simulink model "Final_Project_EEM_Particle_SIM"  (R2020a)
settings: Solver=ode45  StartTime=0  StopTime=t_runtime  FixedStep=clockt/4  RelTol=1e-3  AbsTol=1e-6
PreLoadFcn:
  | run('Final_Project_EEM_SIM_init_params.m');
StopFcn:
  | run('Particle_Simulation_Run_Plots_EEM.m');
undefined symbols (not defined in the file or in its folder): alph1, alphs1, alphsu, alphsv, alphu, alphv, clockt, DB, deg, delt, e0_0, e1_0, e2_0, e3_0, euler_0, f_moon, Force, Inertia_0, L_arm, lla_0, mass_0, Newton, omega_moon, pqr_0, r_moon_eq, rad, Raphson, s, tmin, vel_0
libraries: sharedtransform x5, sharedutil x5, aerolibtransform2 x4, shared6dofsys x3, aerolibconvert2 x3, vrlib x2, aerolibutil x1, aerolibgravity2 x1, aero_libdap x1
(part 1 of 2)
CloseFcn:
  | h=findobj('type','figure','Name','aero_dap3dof');if ~isempty(h);close(h);end
Description:
  | Apollo Lunar Module Digital Autopilot
  | 
  | This model was featured in "Fly Me to the Moon - Then and Now", the story of the digital
  | autopilot in the Lunar Module from the Summer 1999 issue of "MATLAB(R) News & Notes".
  | Double click on the link in the model to view the article online over the Internet.
settings Model: RequirementInfo=9  ExtModeTrigMode=oneshot  ExtModeArmWhenConnect=off  ExtModeAutoUpdateStatusClock=off  Creator=The MathWorks, Inc.  LastModifiedBy=emcneil
settings SolverCC: AutoScaleAbsTol=off
settings DataIOCC: SaveFormat=Array  ReturnWorkspaceOutputs=off  SignalLoggingName=logsOut
settings OptimizationCC: BlockReduction=off  ExpressionDepthLimit=2147483647  InitFltsAndDblsToZero=on
settings DebuggingCC: SaveWithParameterizedLinksMsg=none  SignalResolutionControl=TryResolveAllWithWarning  MultiTaskDSMMsg=warning  MultiTaskCondExecSysMsg=none  SigSpecEnsureSampleTimeMsg=none  FcnCallInpInsideContextMsg=warning  StateNameClashWarn=warning  SFUnexpectedBacktrackingDiag=warning  SFNoUnconditionalDefaultTransitionDiag=warning  SFExecutionAtInitializationDiag=none  ArithmeticOperatorsInVariantConditions=warning
settings HardwareCC: ProdBitPerPointer=32  ProdBitPerSizeT=32  ProdBitPerPtrDiffT=32  ProdLargestAtomicFloat=None  ProdIntDivRoundTo=Undefined  ProdEndianess=Unspecified  ProdWordSize=32  ProdHWDeviceType=Specified
settings ModelReferenceCC: PropagateSignalLabelsOutOfModel=off
settings SFSimCC: SimUseLocalCustomCode=off  SimParseCustomCode=off  CustomCodeUndefinedFunction=UseInterfaceOnly
settings RTWCC: Description=Generic Real-Time Target  RTWUseLocalCustomCode=off
settings CodeAppCC: StateflowObjectComments=on
settings GRTTargetCC: TargetLangStandard=C89/C90 (ANSI)
settings ConfigComp: CovMetricSettings=d  CovHtmlReporting=on  CovSaveCumulativeToWorkspaceVar=on  CovSaveSingleToWorkspaceVar=on  CovExternalEMLEnable=off

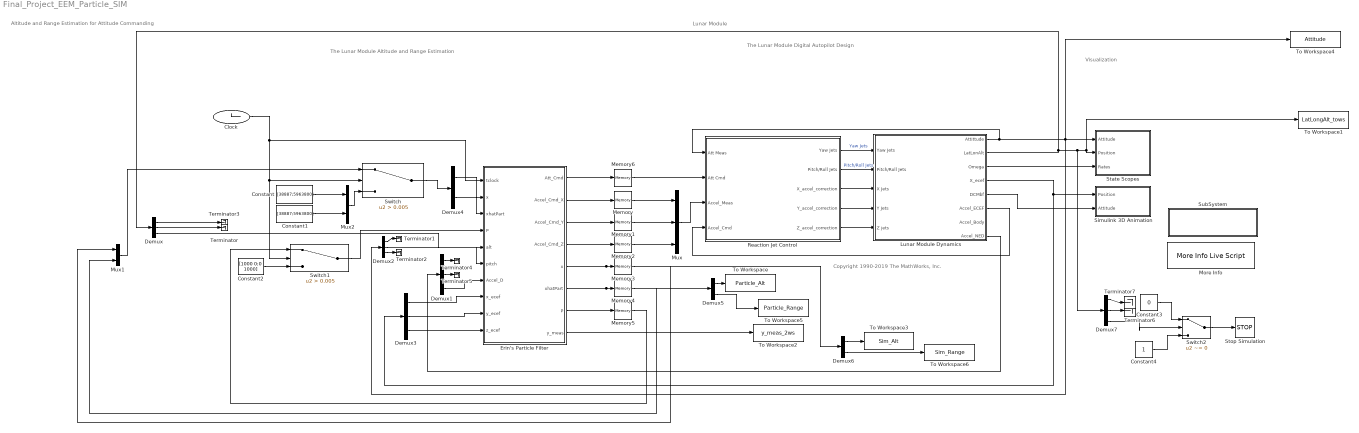
== system Final_Project_EEM_Particle_SIM ==
  note: Lunar Module
  note: Visualization
  note: The Lunar Module Digital Autopilot Design
  note: Copyright 1990-2019 The MathWorks, Inc.
  note: Altitude and Range Estimation for Attitude Commanding
  note: The Lunar Module Altitude and Range Estimation
  Clock : Clock
  Constant : Constant  Value=[38887;5963800]  VectorParams1D=off
  Constant1 : Constant  Value=[38887;5963800]  VectorParams1D=off
  Constant2 : Constant  Value=[1000 0;0 1000]  VectorParams1D=off
  Constant3 : Constant  Value=0
  Constant4 : Constant
  Demux{,1..3,7} (5 alike) : Demux  Outputs=3
  Demux4 : Demux  Outputs=2
  Demux5 : Demux  Outputs=2
  Demux6 : Demux  Outputs=2
  Erin's Particle Filter : MATLAB Function  Description=|  TreatAsAtomicUnit=on
      | This matlab function block was originally created by Erin McNeil 
      | (emcneil8@gatech.edu)for the AE6505 course at Georgia Institute of 
      | Technology Spring 2024 Semester. 
      | The Particle Filter implemented in this block estimates the altitude
      | and range of the vehicle from the Sea of Tranquility landing site on the Lunar
      | Surface and makes an optimal estimate of the values based on the plant model
      | dynamics as well as nonlinear noisy measurement updates. It additionally
      | sends out Pitch angle commands at prescribed altitudes to the 3-DOF 
      | autopilot to acheive an almost upright position at touchdown to the 
      | lunar surface.
  Lunar Module Dynamics : Subsystem
      mask Display: image('aeroLunarModule.jpg');
  Memory{,1..2,6} (4 alike) : Memory  InitialCondition=[0]
  Memory3 : Memory  InitialCondition=[0;0]
  Memory4 : Memory  InitialCondition=[0;0]
  Memory5 : Memory  InitialCondition=[0 0;0 0]
  More Info : aero_libdap/More Info Live Script  SystemSampleTime=-1  Latency=0  AutoFrameSizeCalculation=off
      settings: SourceProductBaseCode=SL
  Mux : Mux  Inputs=3
  Mux1 : Mux  Inputs=2
  Mux2 : Mux  Inputs=2
  Reaction Jet Control : Subsystem
      mask Display: image('aeroLunarReactionJets.png');
  Simulink 3D Animation : Subsystem  mask(Set Animation Properties){enableVis=on, visSampleTime=1}
      mask prompts: enableVis "Enable visualization with Simulink 3D Animation"; visSampleTime "Animation refresh rate:"
      mask help:
      | Change visualization properties used by Simulink 3D Animation. These settings are graphical only and do not affect simulation behavior.
      |
      | Hover over a dialog box for an explanation of the property.
      settings: OpenFcn=|
      | if ~builtin('license','test','virtual_reality_toolbox')
      |     set_param(gcb, 'enableVis', 'off');
      | end
      | open_system(gcb,'mask');
      mask Callback enableVis:
      | if strcmp(get_param(gcb,'enableVis'), 'on')
      |     enable = {'on', 'on'};
      |     set_param(gcb, 'Commented', 'off');
      | else
      |     enable = {'on', 'off'};
      |     set_param(gcb, 'Commented', 'on');
      | end
      | set_param(gcb,'MaskEnables', enable);
      | clear enable
      mask DialogControl vrOpenBtn Prompt: Open Simulink 3D Animation window
      mask DialogControl vrOpenBtn Callback: vrmfunc('FnOpen',getSimulinkBlockHandle([gcb '/VR Sink']));
      mask DialogControl visSampleTime Tooltip: <html>Sample time of animation window. Use this property to effectively speed up or slow down the animation. For example, a sample time of 1 causes the animation to update at every simulation time step. For a sample time of 20, the visualization will update every twentieth simulation time step. Maximum value is 1000.</html>
      mask Display:
      | port_label('input', 1, 'X_{MCMF}','texmode','on')
      | port_label('input', 2, 'DCM_{MCMF2Body}','texmode','on')
  State Scopes : Subsystem
  Stop Simulation : Stop
  SubSystem : Subsystem
      mask init:
      | dispstr = sprintf('Read the technical\narticle for this model.\n(Double-click)');
      settings: OpenFcn=web('https://www.mathworks.com/company/newsletters/articles/the-apollo-11-moon-landing-spacecraft-design-then-and-now.html')
      mask Display: disp(dispstr)
  Switch : Switch  Criteria=u2 > Threshold  Threshold=0.005
  Switch1 : Switch  Criteria=u2 > Threshold  Threshold=0.005
  Switch2 : Switch  Criteria=u2 ~= 0
  Terminator{,1..7} (8 alike) : Terminator
  To Workspace : ToWorkspace  VariableName=Particle_Alt  SampleTime=0.1
      settings: Save2DSignal=2-D array (concatenate along first dimension)
  To Workspace1 : ToWorkspace  VariableName=LatLongAlt_tows  SampleTime=0.1
      settings: Save2DSignal=2-D array (concatenate along first dimension)
  To Workspace2 : ToWorkspace  VariableName=y_meas_2ws  SampleTime=0.1
      settings: Save2DSignal=2-D array (concatenate along first dimension)
  To Workspace3 : ToWorkspace  VariableName=Sim_Alt  SampleTime=0.1
      settings: Save2DSignal=2-D array (concatenate along first dimension)
  To Workspace4 : ToWorkspace  VariableName=Attitude  SampleTime=0.1
      settings: Save2DSignal=2-D array (concatenate along first dimension)
  To Workspace5 : ToWorkspace  VariableName=Particle_Range  SampleTime=0.1
      settings: Save2DSignal=2-D array (concatenate along first dimension)
  To Workspace6 : ToWorkspace  VariableName=Sim_Range  SampleTime=0.1
      settings: Save2DSignal=2-D array (concatenate along first dimension)
  wires:
  Lunar Module Dynamics/3(Omega) -> State Scopes/3(Rates)
  Reaction Jet Control/2(Pitch/Roll Jets) -> Lunar Module Dynamics/2(Pitch/Roll Jets)  "Pitch/Roll Jets"
  Reaction Jet Control/1(Yaw Jets) -> Lunar Module Dynamics/1(Yaw Jets)  "Yaw Jets"
  Lunar Module Dynamics/4(X_ecef) -> Demux3/1, Simulink 3D Animation/1(Position)
  Lunar Module Dynamics/5(DCMbf) -> Simulink 3D Animation/2(Attitude)
  Lunar Module Dynamics/6(Accel_ECEF) -> Reaction Jet Control/4(Accel_Cmd)
  Mux/1 -> Reaction Jet Control/3(Accel_Meas)
  Demux/3 -> Erin's Particle Filter/5(alt)
  Demux/2 -> Terminator/1
  Demux1/3 -> Erin's Particle Filter/7(Accel_D)
  Demux2/2 -> Erin's Particle Filter/6(pitch)
  Demux2/1 -> Terminator1/1
  Demux2/3 -> Terminator2/1
  Demux/1 -> Terminator3/1
  Demux3/1 -> Erin's Particle Filter/8(x_ecef)
  Demux3/2 -> Erin's Particle Filter/9(y_ecef)
  Demux3/3 -> Erin's Particle Filter/10(z_ecef)
  Erin's Particle Filter/3(Accel_Cmd_Y) -> Memory1/1
  Erin's Particle Filter/2(Accel_Cmd_X) -> Memory/1
  Erin's Particle Filter/4(Accel_Cmd_Z) -> Memory2/1
  Reaction Jet Control/3(X_accel_correction) -> Lunar Module Dynamics/3(X Jets)
  Reaction Jet Control/4(Y_accel_correction) -> Lunar Module Dynamics/4(Y Jets)
  Reaction Jet Control/5(Z_accel_correction) -> Lunar Module Dynamics/5(Z jets)
  Memory/1 -> Mux/1
  Memory1/1 -> Mux/2
  Memory2/1 -> Mux/3
  Clock/1 -> Erin's Particle Filter/1(tclock), Switch1/2, Switch/2
  Mux1/1 -> Switch/1
  Switch/1 -> Demux4/1
  Memory3/1 -> Mux1/1
  Memory4/1 -> Mux1/2
  Memory5/1 -> Switch1/1
  Mux2/1 -> Switch/3
  Constant2/1 -> Switch1/3
  Constant/1 -> Mux2/1
  Switch1/1 -> Erin's Particle Filter/4("P ")
  Constant1/1 -> Mux2/2
  Demux4/1 -> Erin's Particle Filter/2("x ")
  Demux4/2 -> Erin's Particle Filter/3("xhatPart ")
  Erin's Particle Filter/6(xhatPart) -> Demux5/1, Memory4/1
  Erin's Particle Filter/1(Att_Cmd) -> Memory6/1
  Memory6/1 -> Reaction Jet Control/2(Att Cmd)
  Erin's Particle Filter/8(y_meas) -> To Workspace2/1
  Erin's Particle Filter/5(x) -> Demux6/1, Memory3/1
  Demux5/1 -> To Workspace/1
  Demux5/2 -> To Workspace5/1
  Demux6/1 -> To Workspace3/1
  Demux6/2 -> To Workspace6/1
  Constant3/1 -> Switch2/1
  Constant4/1 -> Switch2/3
  Demux7/3 -> Switch2/2
  Demux7/2 -> Terminator6/1
  Demux7/1 -> Terminator7/1
  Switch2/1 -> Stop Simulation/1
  Lunar Module Dynamics/8(Accel_NED) -> Demux1/1
  Lunar Module Dynamics/2(LatLonAlt) -> To Workspace1/1, State Scopes/2(Position), Demux7/1, Demux/1
  Erin's Particle Filter/7(P) -> Memory5/1
  Lunar Module Dynamics/1(Attittude) -> Reaction Jet Control/1(Att Meas), To Workspace4/1, State Scopes/1(Attitude), Demux2/1
  Demux1/1 -> Terminator4/1
  Demux1/2 -> Terminator5/1

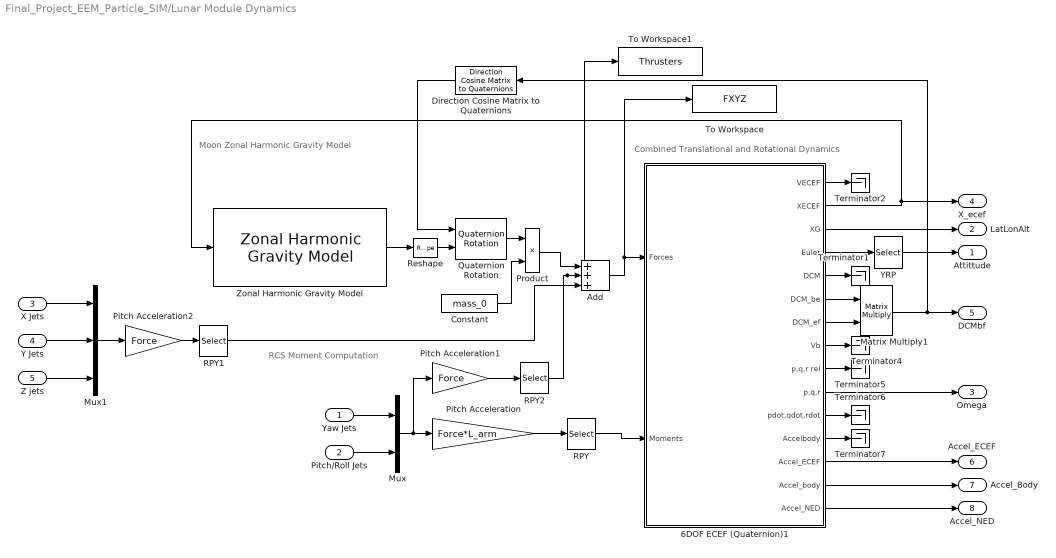
== system Final_Project_EEM_Particle_SIM/Lunar Module Dynamics ==
  note: RCS Moment Computation
  note: Combined Translational and Rotational Dynamics
  note: Moon Zonal Harmonic Gravity Model
  Yaw Jets : Inport  Unit=lbf
  Pitch/Roll Jets : Inport  Port=2  Unit=lbf
  X Jets : Inport  Port=3  Unit=lbf
  Y Jets : Inport  Port=4  Unit=lbf
  Z jets : Inport  Port=5  Unit=lbf
  6DOF ECEF (Quaternion)1 : Subsystem  AncestorBlock=aerolib6dof2/6DOF ECEF (Quaternion)  mask(6DOF EoM (ECEF)){units=English (Velocity in ft/s), mtype=Fixed, xg_0=lla_0, Vm_0=vel_0, eul_0=euler_0*pi/180, pm_0=pqr_0*pi/180, mass_0=mass_0, mass_e=0.5, mass_f=2.0, inertia=Inertia_0, inertia_e=eye(3), inertia_f=2*eye(3), vre_flag=on, abi_flag=off, ptype=Custom, R=r_moon_eq, F=f_moon, w_E=omega_moon, angle_in=Internal, LG0=0, quat_statename='', pm_statename='', Vm_statename='', posECEF_statename='', posECI_statename='', LG_statename='', mass_statename=''}
      mask prompts: units "aeroblks:aeroblk6dofbody:block6DOFEoMECEFParamUnits"; mtype "aeroblks:aeroblk6dofbody:block6DOFEoMECEFParamMasstype"; xg_0 "aeroblks:aeroblk6dofbody:block6DOFEoMECEFParamInitialpositioningeodeticlatitudelongitudealtitudemulh"; Vm_0 "aeroblks:aeroblk6dofbody:block6DOFEoMECEFParamInitialvelocityinbodyaxesUvw"; eul_0 "aeroblks:aeroblk6dofbody:block6DOFEoMECEFParamInitialEulerorientationrollpitchyaw"; pm_0 "aeroblks:aeroblk6dofbody:block6DOFEoMECEFParamInitialbodyrotationratespqr"; mass_0 "aeroblks:aeroblk6dofbody:block6DOFEoMECEFParamInitialmass"; mass_e "aeroblks:aeroblk6dofbody:block6DOFEoMECEFParamEmptymass"; mass_f "aeroblks:aeroblk6dofbody:block6DOFEoMECEFParamFullmass"; inertia "aeroblks:aeroblk6dofbody:block6DOFEoMECEFParamInertia"; inertia_e "aeroblks:aeroblk6dofbody:block6DOFEoMECEFParamEmptyinertiamatrix"; inertia_f "aeroblks:aeroblk6dofbody:block6DOFEoMECEFParamFullinertiamatrix"; vre_flag "aeroblks:aeroblk6dofbody:block6DOFEoMECEFParamIncludemassflowrelativevelocity"; abi_flag "aeroblks:aeroblk6dofecef:inertialAccelFlag"; ptype "aeroblks:aeroblk6dofbody:block6DOFEoMECEFParamPlanetmodel"; R "aeroblks:aeroblk6dofbody:block6DOFEoMECEFParamEquatorialradius"; F "aeroblks:aeroblk6dofbody:block6DOFEoMECEFParamFlattening"; w_E "aeroblks:aeroblk6dofbody:block6DOFEoMECEFParamRotationalrateradsec"; angle_in "aeroblks:aeroblk6dofbody:block6DOFEoMECEFParamCelestiallongitudeofGreenwichsource"; LG0 "aeroblks:aeroblk6dofbody:block6DOFEoMECEFParamCelestiallongitudeofGreenwichdeg"; quat_statename "aeroblks:aeroblk6dofbody:block6DOFEoMECEFStateNameQuaternions"; pm_statename "aeroblks:aeroblk6dofbody:block6DOFEoMECEFStateNameRotationRates"; Vm_statename "aeroblks:aeroblk6dofbody:block6DOFEoMECEFStateNameVelocity"; posECEF_statename "aeroblks:aeroblk6dofbody:block6DOFEoMECEFStateNameECEFPosition"; posECI_statename "aeroblks:aeroblk6dofbody:block6DOFEoMECEFStateNameECIPosition"; LG_statename "aeroblks:aeroblk6dofbody:block6DOFEoMECEFStateNameCelestLon"; mass_statename "aeroblks:aeroblk6dofbody:block6DOFEoMECEFStateNameMass"
      mask help: aeroblks:aeroblk6dofbody:block6DOFEoMECEFDesc
      mask init:
      | [ports]=aeroicon('aeroblk6dofecef','icon');
      mask Help: eval('asbhelp(''sixdof_ecef_quaternion'')');
      mask TypeOptions units: aeroblks:aeroblk6dofbody:block6DOFEoMECEFParamComboMetricMKS | aeroblks:aeroblk6dofbody:block6DOFEoMECEFParamComboEnglishVelocityinfts | aeroblks:aeroblk6dofbody:block6DOFEoMECEFParamComboEnglishVelocityinkts
      mask TypeOptions mtype: aeroblks:aeroblk6dofbody:block6DOFEoMECEFParamComboFixed | aeroblks:aeroblk6dofbody:block6DOFEoMECEFParamComboSimpleVariable | aeroblks:aeroblk6dofbody:block6DOFEoMECEFParamComboCustomVariable
      mask Callback mtype: aeroicon('aeroblk6dofecef');
      mask TypeOptions ptype: aeroblks:aeroblk6dofbody:block6DOFEoMECEFParamComboCustom | aeroblks:aeroblk6dofbody:block6DOFEoMECEFParamComboEarthWGS84
      mask Callback ptype: aeroicon('aeroblk6dofecef');
      mask TypeOptions angle_in: aeroblks:aeroblk6dofbody:block6DOFEoMECEFParamComboInternal | aeroblks:aeroblk6dofbody:block6DOFEoMECEFParamComboExternal
      mask Callback angle_in: aeroicon('aeroblk6dofecef');
      mask DialogControl Container4 Prompt: aeroblks:aeroblk6dofbody:block6DOFEoMECEFMainTab
      mask DialogControl units Prompt: Units:
      mask DialogControl mtype Prompt: Mass type:
      mask DialogControl xg_0 Prompt: Initial position in geodetic latitude, longitude, altitude [mu,l,h]:
      mask DialogControl Vm_0 Prompt: Initial velocity in body axes [U,v,w]:
      mask DialogControl eul_0 Prompt: Initial Euler orientation [roll, pitch, yaw]:
      mask DialogControl pm_0 Prompt: Initial body rotation rates [p,q,r]:
      mask DialogControl mass_0 Prompt: Initial mass:
      mask DialogControl mass_e Prompt: Empty mass:
      mask DialogControl mass_f Prompt: Full mass:
      mask DialogControl inertia Prompt: Inertia:
      mask DialogControl inertia_e Prompt: Empty inertia matrix:
      mask DialogControl inertia_f Prompt: Full inertia matrix:
      mask DialogControl vre_flag Prompt: Include mass flow relative velocity
      mask DialogControl abi_flag Prompt: Include inertial acceleration
      mask DialogControl Container5 Prompt: aeroblks:aeroblk6dofbody:block6DOFEoMECEFPlanetTab
      mask DialogControl ptype Prompt: Planet model:
      mask DialogControl R Prompt: Equatorial radius:
      mask DialogControl F Prompt: Flattening:
      mask DialogControl w_E Prompt: Rotational rate [rad/sec]:
      mask DialogControl angle_in Prompt: Celestial longitude of Greenwich source:
      mask DialogControl LG0 Prompt: Celestial longitude of Greenwich [deg]:
      mask DialogControl Container6 Prompt: aeroblks:aeroblk6dofbody:block6DOFEoMECEFStateAttributesTab
      mask DialogControl Container7 Prompt: aeroblks:aeroblk6dofbody:block6DOFEoMECEFStateNamesGroup
      mask DialogControl quat_statename Prompt: Quaternion vector: e.g., {'qr', 'qi', 'qj', 'qk'}
      mask DialogControl pm_statename Prompt: Body rotation rates: e.g., {'p', 'q', 'r'}
      mask DialogControl Vm_statename Prompt: Velocity: e.g., {'U', 'v', 'w'}
      mask DialogControl posECEF_statename Prompt: ECEF position: e.g., {'Xecef', 'Yecef', 'Zecef'}
      mask DialogControl posECI_statename Prompt: Inertial position: e.g., {'Xeci', 'Yeci', 'Zeci'}
      mask DialogControl LG_statename Prompt: Celestial longitude of Greenwich: e.g., 'LG'
      mask DialogControl mass_statename Prompt: Mass: e.g., 'mass'
      mask Display:
      | port_label(ports(1).type,ports(1).port,ports(1).txt,'texmode','on');
      | port_label(ports(2).type,ports(2).port,ports(2).txt,'texmode','on');
      | port_label(ports(3).type,ports(3).port,ports(3).txt,'texmode','on');
      | port_label(ports(4).type,ports(4).port,ports(4).txt,'texmode','on');
      | port_label(ports(5).type,ports(5).port,ports(5).txt,'texmode','on');
      | port_label(ports(6).type,ports(6).port,ports(6).txt,'texmode','on');
      | port_label(ports(7).type,ports(7).port,ports(7).txt,'texmode','on');
      | port_label(ports(8).type,ports(8).port,ports(8).txt,'texmode','on');
      | port_label(ports(9).type,ports(9).port,ports(9).txt,'texmode','on');
      | port_label(ports(10).type,ports(10).port,ports(10).txt,'texmode','on');
      | port_label(ports(11).type,ports(11).port,ports(11).txt,'texmode','on');
      | port_label(ports(12).type,ports(12).port,ports(12).txt,'texmode','on');
      | port_label(ports(13).type,ports(13).port,ports(13).txt,'texmode','on');
      | port_label(ports(14).type,ports(14).port,ports(14).txt,'texmode','on');
      | port_label(ports(15).type,ports(15).port,ports(15).txt,'texmode','on');
      | port_label(ports(16).type,ports(16).port,ports(16).txt,'texmode','on');
      | port_label(ports(17).type,ports(17).port,ports(17).txt,'texmode','on');
      | port_label(ports(18).type,ports(18).port,ports(18).txt,'texmode','on');
      | port_label(ports(19).type,ports(19).port,ports(19).txt,'texmode','on');
      | port_label(ports(20).type,ports(20).port,ports(20).txt,'texmode','on');
      | port_label(ports(21).type,ports(21).port,ports(21).txt,'texmode','on');
      | port_label(ports(22).type,ports(22).port,ports(22).txt,'texmode','on');
  Add : Sum  Inputs=+++
  Constant : Constant  Value=mass_0
  Direction Cosine Matrix to Quaternions : sharedtransform/Direction Cosine Matrix  to Quaternions  aMode=0  action=None  tolerance=eps(2)
      settings: SourceProductBaseCode=AE,PW,MT,VE,VP
  Matrix Multiply1 : Product  Multiplication=Matrix(*)
  Mux : Mux  Inputs=2
  Mux1 : Mux  Inputs=3
  Pitch Acceleration : Gain  Gain=Force*L_arm  SaturateOnIntegerOverflow=on  OutDataTypeStr=Inherit: Same as input  ParamDataTypeStr=Inherit: Same as input
  Pitch Acceleration1 : Gain  Gain=Force  SaturateOnIntegerOverflow=on  OutDataTypeStr=Inherit: Same as input  ParamDataTypeStr=Inherit: Same as input
  Pitch Acceleration2 : Gain  Gain=Force  SaturateOnIntegerOverflow=on  OutDataTypeStr=Inherit: Same as input  ParamDataTypeStr=Inherit: Same as input
  Product : Product
  Quaternion Rotation : aerolibutil/Quaternion Rotation
  RPY : Selector  InputPortWidth=3  IndexOptions=Index vector (dialog)  Indices=[2 3 1]  OutputSizes=1
  RPY1 : Selector  InputPortWidth=3  IndexOptions=Index vector (dialog)  Indices=[1 2 3]  OutputSizes=1
  RPY2 : Selector  InputPortWidth=3  IndexOptions=Index vector (dialog)  Indices=[2 3 1]  OutputSizes=1
  Reshape : Reshape
  Terminator{1..2,4..7} (6 alike) : Terminator
  To Workspace : ToWorkspace  VariableName=FXYZ  SampleTime=0.1
      settings: Save2DSignal=2-D array (concatenate along first dimension)
  To Workspace1 : ToWorkspace  VariableName=Thrusters  SampleTime=0.1
      settings: Save2DSignal=2-D array (concatenate along first dimension)
  YRP : Selector  InputPortWidth=3  IndexOptions=Index vector (dialog)  Indices=[3 1 2]  OutputSizes=1
  Zonal Harmonic Gravity Model : aerolibgravity2/Zonal Harmonic Gravity Model  units=English  degree=2  action=Warning  ptype=Moon  R=5702099.7375  GM=173140712687447.5  jvalue=[2.0270000e-04]
      settings: SourceProductBaseCode=AE
  Attittude : Outport  Unit=rad  VectorParamsAs1DForOutWhenUnconnected=off
  LatLonAlt : Outport  Port=2  VectorParamsAs1DForOutWhenUnconnected=off
  Omega : Outport  Port=3  Unit=rad/s  VectorParamsAs1DForOutWhenUnconnected=off
  X_ecef : Outport  Port=4  Unit=ft  VectorParamsAs1DForOutWhenUnconnected=off
  DCMbf : Outport  Port=5  VectorParamsAs1DForOutWhenUnconnected=off
  Accel_ECEF : Outport  Port=6  Unit=ft/sec^2  VectorParamsAs1DForOutWhenUnconnected=off
  Accel_Body : Outport  Port=7  Unit=ft/sec^2  VectorParamsAs1DForOutWhenUnconnected=off
  Accel_NED : Outport  Port=8  Unit=ft/sec^2  VectorParamsAs1DForOutWhenUnconnected=off
  wires:
  Yaw Jets/1 -> Mux/1
  Mux/1 -> Pitch Acceleration1/1, Pitch Acceleration/1
  6DOF ECEF (Quaternion)1/4(Euler) -> YRP/1
  6DOF ECEF (Quaternion)1/10(p,q,r) -> Omega/1
  Matrix Multiply1/1 -> Direction Cosine Matrix to Quaternions/1, DCMbf/1
  6DOF ECEF (Quaternion)1/6(DCM_be) -> Matrix Multiply1/1
  6DOF ECEF (Quaternion)1/7(DCM_ef) -> Matrix Multiply1/2
  Zonal Harmonic Gravity Model/1 -> Reshape/1
  Quaternion Rotation/1 -> Product/1
  Reshape/1 -> Quaternion Rotation/2
  Direction Cosine Matrix to Quaternions/1 -> Quaternion Rotation/1
  6DOF ECEF (Quaternion)1/1(VECEF) -> Terminator2/1
  6DOF ECEF (Quaternion)1/5(DCM) -> Terminator1/1
  6DOF ECEF (Quaternion)1/2(XECEF) -> Zonal Harmonic Gravity Model/1, X_ecef/1
  6DOF ECEF (Quaternion)1/9(p,q,r rel) -> Terminator5/1
  6DOF ECEF (Quaternion)1/8(Vb) -> Terminator4/1
  6DOF ECEF (Quaternion)1/11(pdot,qdot,rdot) -> Terminator6/1
  6DOF ECEF (Quaternion)1/12(Accelbody) -> Terminator7/1
  6DOF ECEF (Quaternion)1/3(XG) -> LatLonAlt/1
  Constant/1 -> Product/2
  Product/1 -> Add/1
  Pitch Acceleration/1 -> RPY/1
  RPY/1 -> 6DOF ECEF (Quaternion)1/2(Moments)
  YRP/1 -> Attittude/1
  Pitch/Roll Jets/1 -> Mux/2
  6DOF ECEF (Quaternion)1/13(Accel_ECEF) -> Accel_ECEF/1
  6DOF ECEF (Quaternion)1/14(Accel_body) -> Accel_Body/1
  Add/1 -> To Workspace/1, 6DOF ECEF (Quaternion)1/1(Forces)
  RPY2/1 -> To Workspace1/1, Add/2
  Pitch Acceleration1/1 -> RPY2/1
  X Jets/1 -> Mux1/1
  Y Jets/1 -> Mux1/2
  Z jets/1 -> Mux1/3
  Mux1/1 -> Pitch Acceleration2/1
  Pitch Acceleration2/1 -> RPY1/1
  RPY1/1 -> Add/3
  6DOF ECEF (Quaternion)1/15(Accel_NED) -> Accel_NED/1

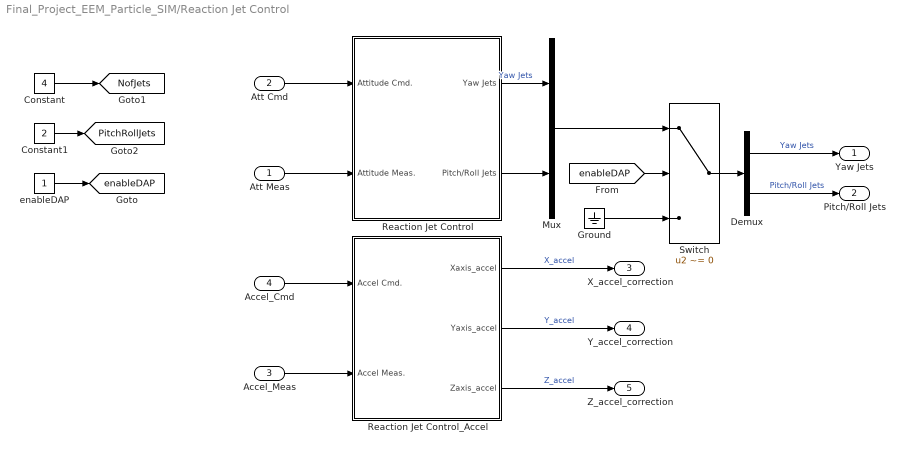
== system Final_Project_EEM_Particle_SIM/Reaction Jet Control ==
  Att Meas : Inport
  Att Cmd : Inport  Port=2
  Accel_Meas : Inport  Port=3
  Accel_Cmd : Inport  Port=4
  Constant : Constant  Value=4
  Constant1 : Constant  Value=2
  Demux : Demux  Outputs=[1 2]
  Ground : Ground
  Mux : Mux  Inputs=2
  Reaction Jet Control : Subsystem  AncestorBlock=aero_librcs/Reaction Jet Control
  Reaction Jet Control_Accel : Subsystem  AncestorBlock=aero_librcs/Reaction Jet Control
  Switch : Switch  Criteria=u2 ~= 0
  enableDAP : Constant
  Yaw Jets : Outport  VectorParamsAs1DForOutWhenUnconnected=off
  Pitch/Roll Jets : Outport  Port=2  VectorParamsAs1DForOutWhenUnconnected=off
  X_accel_correction : Outport  Port=3
  Y_accel_correction : Outport  Port=4
  Z_accel_correction : Outport  Port=5
  tag scope: NofJets=global, PitchRollJets=global, enableDAP=global
  wires:
  Att Cmd/1 -> Reaction Jet Control/1(Attitude Cmd.)
  Att Meas/1 -> Reaction Jet Control/2(Attitude Meas.)
  Demux/1 -> Yaw Jets/1  "Yaw Jets"
  Demux/2 -> Pitch/Roll Jets/1  "Pitch/Roll Jets"
  Ground/1 -> Switch/3
  Reaction Jet Control/1(Yaw Jets) -> Mux/1  "Yaw Jets"
  [enableDAP] -> Switch/2
  Mux/1 -> Switch/1
  Reaction Jet Control/2(Pitch/Roll Jets) -> Mux/2
  Switch/1 -> Demux/1
  Accel_Meas/1 -> Reaction Jet Control_Accel/2(Accel Meas.)
  Accel_Cmd/1 -> Reaction Jet Control_Accel/1(Accel Cmd.)
  Reaction Jet Control_Accel/1(Xaxis_accel) -> X_accel_correction/1  "X_accel"
  Reaction Jet Control_Accel/2(Yaxis_accel) -> Y_accel_correction/1  "Y_accel"
  Reaction Jet Control_Accel/3(Zaxis_accel) -> Z_accel_correction/1  "Z_accel"
  Constant1/1 -> [PitchRollJets]
  enableDAP/1 -> [enableDAP]
  Constant/1 -> [NofJets]

== system Final_Project_EEM_Particle_SIM/Simulink 3D Animation ==
  Position : Inport
  Attitude : Inport  Port=2
  Convert to VR Units : Subsystem
  VR Sink : vrlib/VR Sink  InstantiateOnLoad=on  SampleTime=visSampleTime  ViewEnable=on  RemoteChange=off  RemoteView=off  FieldsWritten=LSAM.rotation.4.1.1.double#LSAM.translation.3.1.1.double  WorldFileName=Lander_Moon180_1.wrl  WorldDescription=Apollo Lunar Module Descent Animation  AutoView=on  VideoDimensions=[]  AllowVariableSize=off
  wires:
  Attitude/1 -> Convert to VR Units/1(Att)
  Position/1 -> Convert to VR Units/2(Pos)
  Convert to VR Units/1(attVR) -> VR Sink/1
  Convert to VR Units/2(posVR) -> VR Sink/2

== system Final_Project_EEM_Particle_SIM/State Scopes ==
  Attitude : Inport
  Position : Inport  Port=2
  Rates : Inport  Port=3
  Angle Conversion : aerolibconvert2/Angle Conversion  IU=rad  OU=deg
  Angular Velocity Conversion : aerolibconvert2/Angular Velocity Conversion  IU=rad/s  OU=deg/s
  Body Attitude : Scope
  Body Rates : Scope
  Demux : Demux  Outputs=[2 1]
  LatLonAlt : Scope  NumInputPorts=2
  RPY : Selector  InputPortWidth=3  IndexOptions=Index vector (dialog)  Indices=[2 3 1]  OutputSizes=1
  Signal Specification : SignalSpecification  Unit=deg
  Signal Specification1 : SignalSpecification  Unit=ft
  wires:
  Attitude/1 -> RPY/1
  Rates/1 -> Angular Velocity Conversion/1
  Demux/2 -> Signal Specification1/1
  Demux/1 -> Signal Specification/1
  Position/1 -> Demux/1
  Angle Conversion/1 -> Body Attitude/1
  Angular Velocity Conversion/1 -> Body Rates/1
  Signal Specification/1 -> LatLonAlt/1
  Signal Specification1/1 -> LatLonAlt/2
  RPY/1 -> Angle Conversion/1

== system Final_Project_EEM_Particle_SIM/SubSystem ==

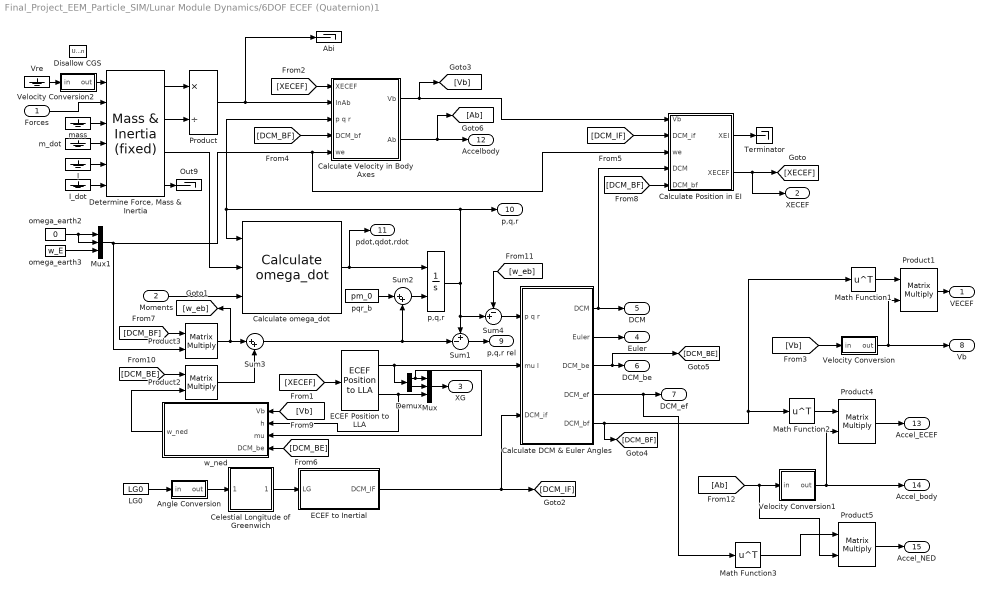
== system Final_Project_EEM_Particle_SIM/Lunar Module Dynamics/6DOF ECEF (Quaternion)1 ==
  Forces : Inport  Unit=lb  PortDimensions=3
  Moments : Inport  Port=2  Unit=lb*ft  PortDimensions=3
  Abi : Terminator
  Angle Conversion : Subsystem
  Calculate DCM & Euler Angles : Subsystem  mask(DCM & Euler Angles (Quaternion)){}
  "Calculate Position in EI " : Subsystem
  Calculate Velocity in Body Axes : Subsystem
  Calculate omega_dot : shared6dofsys/Calculate omega_dot  aMode=aMode
      settings: SourceProductBaseCode=AE,PW,MT,VE,VP
  Celestial Longitude of Greenwich : Subsystem
      mask Display:
      | port_label('input',1,'L_{G}(0)','texmode','on')
      | port_label('output',1,'L_G','texmode','on')
  Demux : Demux  Outputs=2
  "Determine Force, Mass & Inertia" : shared6dofsys/Mass & Inertia (fixed)  aMode=aMode
      settings: SourceProductBaseCode=AE,PW,MT,VE,VP
  Disallow CGS : UnitConfiguration  UnitSystemsStr=English,SI,SI (extended)  AllowAllUnitSystems=off
  ECEF Position to LLA : aerolibtransform2/ECEF Position to LLA  units=Metric (MKS)  ptype=Custom  F=F  R=R
      settings: SourceProductBaseCode=AE
  ECEF to Inertial : Subsystem
  I : Ground
  I_dot : Ground
  LG0 : Constant  Value=LG0  OutDataTypeStr=Inherit: Inherit via back propagation
  Math Function1 : Math  Operator=transpose  SignedPower=on  SaturateOnIntegerOverflow=on
  Math Function2 : Math  Operator=transpose  SignedPower=on  SaturateOnIntegerOverflow=on
  Math Function3 : Math  Operator=transpose  SignedPower=on  SaturateOnIntegerOverflow=on
  Mux : Mux  Inputs=3
  Mux1 : Mux  Inputs=3
  Out9 : Terminator
  Product : Product  Inputs=*/  SaturateOnIntegerOverflow=on  OutDataTypeStr=Inherit: Same as first input
  Product{1..5} (5 alike) : Product  Multiplication=Matrix(*)  RndMeth=Zero
  Sum1 : Sum  Inputs=+-|
  Sum2 : Sum  Inputs=|++
  Sum3 : Sum  Inputs=|++
  Sum4 : Sum  Inputs=-+|
  Terminator : Terminator
  Velocity Conversion : Subsystem
  Velocity Conversion1 : Subsystem
  Velocity Conversion2 : Subsystem
  Vre : Ground
  m_dot : Ground
  mass : Ground
  omega_earth2 : Constant  Value=0
  omega_earth3 : Constant  Value=w_E
  "p,q,r " : Integrator  InitialConditionSource=external  InitialCondition=pm_0  ContinuousStateAttributes=pm_statename
  pqr_b : Constant  Value=pm_0
  w_ned : Subsystem
  VECEF : Outport  Unit=ft/s  VectorParamsAs1DForOutWhenUnconnected=off
  XECEF : Outport  Port=2  Unit=ft  VectorParamsAs1DForOutWhenUnconnected=off
  XG : Outport  Port=3  VectorParamsAs1DForOutWhenUnconnected=off
  Euler : Outport  Port=4  Unit=rad  VectorParamsAs1DForOutWhenUnconnected=off
  DCM : Outport  Port=5  Unit=1  VectorParamsAs1DForOutWhenUnconnected=off
  DCM_be : Outport  Port=6  Unit=1  VectorParamsAs1DForOutWhenUnconnected=off
  DCM_ef : Outport  Port=7  Unit=1  VectorParamsAs1DForOutWhenUnconnected=off
  Vb : Outport  Port=8  Unit=ft/s  VectorParamsAs1DForOutWhenUnconnected=off
  p,q,r rel : Outport  Port=9  Unit=rad/s  VectorParamsAs1DForOutWhenUnconnected=off
  p,q,r : Outport  Port=10  Unit=rad/s  VectorParamsAs1DForOutWhenUnconnected=off
  pdot,qdot,rdot : Outport  Port=11  Unit=rad/s^2  VectorParamsAs1DForOutWhenUnconnected=off
  Accelbody : Outport  Port=12  Unit=ft/s^2  VectorParamsAs1DForOutWhenUnconnected=off
  Accel_ECEF : Outport  Port=13  Unit=ft/sec^2  VectorParamsAs1DForOutWhenUnconnected=off
  Accel_body : Outport  Port=14  Unit=ft/sec^2  VectorParamsAs1DForOutWhenUnconnected=off
  Accel_NED : Outport  Port=15
  wires:
  Calculate DCM & Euler Angles/4(DCM_ef) -> Math Function3/1, DCM_ef/1
  Calculate DCM & Euler Angles/5(DCM_bf) -> [DCM_BF], Math Function1/1, Math Function2/1
  [DCM_BE] -> Product2/1
  Product3/1 -> Sum3/1, [w_eb]
  "Calculate Position in EI "/2(XECEF) -> XECEF/1, [XECEF]
  "Determine Force, Mass & Inertia"/2 -> Product/2
  Calculate DCM & Euler Angles/1(DCM) -> DCM/1, "Calculate Position in EI "/4(DCM)
  Product1/1 -> VECEF/1
  Calculate DCM & Euler Angles/2(Euler) -> Euler/1
  "Determine Force, Mass & Inertia"/3 -> Calculate omega_dot/2
  Calculate DCM & Euler Angles/3(DCM_be) -> [DCM_BE], DCM_be/1
  [XECEF] -> ECEF Position to LLA/1
  Mux/1 -> XG/1
  ECEF Position to LLA/2 -> w_ned/2(h), Mux/3
  ECEF Position to LLA/1 -> Calculate DCM & Euler Angles/2(mu l), Demux/1
  Mux1/1 -> Product3/2, "Calculate Position in EI "/3(we), Calculate Velocity in Body Axes/5(we)
  [XECEF] -> Calculate Velocity in Body Axes/1(XECEF)
  [DCM_IF] -> "Calculate Position in EI "/2(DCM_if)
  [Vb] -> Velocity Conversion/1(in)
  Celestial Longitude of Greenwich/1(Lambda) -> ECEF to Inertial/1(LG)
  ECEF to Inertial/1(DCM_IF) -> Calculate DCM & Euler Angles/3(DCM_if), [DCM_IF]
  pqr_b/1 -> Sum2/1
  Sum3/1 -> Sum1/2, Sum2/2
  [DCM_BF] -> Product3/1
  Sum1/1 -> p,q,r rel/1
  [DCM_BF] -> "Calculate Position in EI "/5(DCM_bf)
  [DCM_BE] -> w_ned/4(DCM_be)
  [Vb] -> w_ned/1(Vb)
  w_ned/1(w_ned) -> Product2/2
  Product2/1 -> Sum3/2
  Sum4/1 -> Calculate DCM & Euler Angles/1(p q r)
  [w_eb] -> Sum4/1
  Velocity Conversion/1(out) -> Vb/1, Product1/2
  I/1 -> "Determine Force, Mass & Inertia"/5
  I_dot/1 -> "Determine Force, Mass & Inertia"/6
  mass/1 -> "Determine Force, Mass & Inertia"/3
  Forces/1 -> "Determine Force, Mass & Inertia"/2
  "Determine Force, Mass & Inertia"/1 -> Product/1
  m_dot/1 -> "Determine Force, Mass & Inertia"/4
  "Determine Force, Mass & Inertia"/4 -> Out9/1
  [DCM_BF] -> Calculate Velocity in Body Axes/4(DCM_bf)
  Calculate Velocity in Body Axes/1(Vb) -> [Vb], "Calculate Position in EI "/1(Vb)
  "Calculate Position in EI "/1(XEI) -> Terminator/1
  Math Function1/1 -> Product1/1
  LG0/1 -> Angle Conversion/1(in)
  Moments/1 -> Calculate omega_dot/3
  Demux/2 -> Mux/2
  Demux/1 -> Mux/1, w_ned/3(mu)
  "p,q,r "/1 -> Sum1/1, Sum4/2, p,q,r/1, Calculate omega_dot/1, Calculate Velocity in Body Axes/3(p q r)
  Calculate omega_dot/1 -> "p,q,r "/1, pdot,qdot,rdot/1
  Sum2/1 -> "p,q,r "/2
  Vre/1 -> Velocity Conversion2/1(in)
  Velocity Conversion2/1(out) -> "Determine Force, Mass & Inertia"/1
  Calculate Velocity in Body Axes/2(Ab) -> [Ab], Accelbody/1
  omega_earth2/1 -> Mux1/2, Mux1/1
  omega_earth3/1 -> Mux1/3
  Angle Conversion/1(out) -> Celestial Longitude of Greenwich/1(Initial Angle)
  Velocity Conversion1/1(out) -> Product4/2, Accel_body/1
  Product4/1 -> Accel_ECEF/1
  Math Function2/1 -> Product4/1
  Product/1 -> Calculate Velocity in Body Axes/2(InAb), Abi/1
  Product5/1 -> Accel_NED/1
  Math Function3/1 -> Product5/1
  [Ab] -> Product5/2, Velocity Conversion1/1(in)

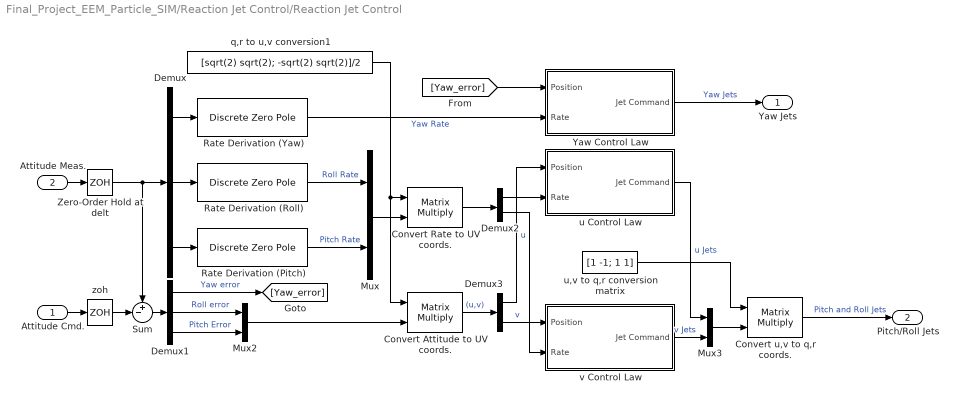
== system Final_Project_EEM_Particle_SIM/Reaction Jet Control/Reaction Jet Control ==
  Attitude Cmd. : Inport  Unit=rad
  Attitude Meas. : Inport  Port=2  Unit=rad
  Convert Attitude to UV coords. : Product  Multiplication=Matrix(*)  InputSameDT=on  RndMeth=Zero  SaturateOnIntegerOverflow=on  OutDataTypeStr=Inherit: Same as first input
  Convert Rate to UV coords. : Product  Multiplication=Matrix(*)  InputSameDT=on  RndMeth=Zero  SaturateOnIntegerOverflow=on  OutDataTypeStr=Inherit: Same as first input
  Convert u,v to q,r coords. : Product  Multiplication=Matrix(*)  InputSameDT=on  RndMeth=Zero  SaturateOnIntegerOverflow=on  OutDataTypeStr=Inherit: Same as first input
  Demux : Demux  Outputs=3
      settings: DisplayOption=none
  Demux1 : Demux  Outputs=3
      settings: DisplayOption=none
  Demux2 : Demux  Outputs=2
      settings: DisplayOption=none
  Demux3 : Demux  Outputs=2
      settings: DisplayOption=none
  Mux : Mux  Inputs=2
  Mux2 : Mux  Inputs=2
  Mux3 : Mux  Inputs=2
  Rate Derivation (Pitch) : DiscreteZeroPole  Poles=[0]  Gain=1/delt  SampleTime=-1
  Rate Derivation (Roll) : DiscreteZeroPole  Poles=[0]  Gain=1/delt  SampleTime=-1
  Rate Derivation (Yaw) : DiscreteZeroPole  Poles=[0]  Gain=1/delt  SampleTime=-1
  Sum : Sum  Inputs=+-|  InputSameDT=on  SaturateOnIntegerOverflow=on  OutDataTypeStr=Inherit: Same as first input
  Yaw Control Law : Subsystem  AncestorBlock=aero_libdap/Yaw Control Law  mask(Control Law){alph=alph1, alphs=alphs1, DB=DB, tmin=tmin, delt=delt}
      mask prompts: alph "Single Jet Accel:"; alphs "Single Jet Switch Curve Accel:"; DB "Dead Band:"; tmin "Min Jet On Time:"; delt "Sample Time:"
      mask help: Implements Control Law for the LM. Works for yaw, u and v jet axes.
  Zero-Order Hold at delt : ZeroOrderHold  SampleTime=delt
  q,r to u,v conversion1 : Constant  Value=[sqrt(2) sqrt(2); -sqrt(2) sqrt(2)]/2  VectorParams1D=off
  u Control Law : Subsystem  AncestorBlock=aero_libdap/Pitch Roll Control Law  mask(Control Law){alph=alphu, alphs=alphsu, DB=DB, tmin=tmin, delt=delt}
      mask prompts: alph "Single Jet Accel:"; alphs "Single Jet Switch Curve Accel:"; DB "Dead Band:"; tmin "Min. Jet On Time:"; delt "Sample Time:"
      mask help: Implements Control Law for the LM. Works for yaw, u and v jet axes.
  u,v to q,r conversion matrix : Constant  Value=[1 -1; 1 1]  VectorParams1D=off
  v Control Law : Subsystem  AncestorBlock=aero_libdap/Pitch Roll Control Law  mask(Control Law){alph=alphv, alphs=alphsv, DB=DB, tmin=tmin, delt=delt}
      mask prompts: alph "Single Jet Accel:"; alphs "Single Jet Switch Curve Accel:"; DB "Dead Band:"; tmin "Min. Jet On Time:"; delt "Sample Time:"
      mask help: Implements Control Law for the LM. Works for yaw, u and v jet axes.
  zoh : ZeroOrderHold  SampleTime=delt
  Yaw Jets : Outport  Unit=lbf  OutputWhenDisabled=reset  InitialOutput=0  VectorParamsAs1DForOutWhenUnconnected=off
  Pitch/Roll Jets : Outport  Port=2  Unit=lbf  OutputWhenDisabled=reset  InitialOutput=0  VectorParamsAs1DForOutWhenUnconnected=off
  wires:
  zoh/1 -> Sum/2
  Zero-Order Hold at delt/1 -> Sum/1, Demux/1
  q,r to u,v conversion1/1 -> Convert Attitude to UV coords./1, Convert Rate to UV coords./1
  Rate Derivation (Pitch)/1 -> Mux/2  "Pitch Rate"
  Rate Derivation (Roll)/1 -> Mux/1  "Roll Rate"
  Demux/2 -> Rate Derivation (Roll)/1
  Demux/3 -> Rate Derivation (Pitch)/1
  Demux/1 -> Rate Derivation (Yaw)/1
  Mux/1 -> Convert Rate to UV coords./2
  Attitude Meas./1 -> Zero-Order Hold at delt/1
  Rate Derivation (Yaw)/1 -> Yaw Control Law/2(Rate)  "Yaw Rate"
  Yaw Control Law/1(Jet Command) -> Yaw Jets/1  "Yaw Jets"
  [Yaw_error] -> Yaw Control Law/1(Position)
  Sum/1 -> Demux1/1
  Demux1/2 -> Mux2/1  "Roll error"
  Demux1/3 -> Mux2/2  "Pitch Error"
  Convert Rate to UV coords./1 -> Demux2/1
  Convert Attitude to UV coords./1 -> Demux3/1  "(u,v)"
  Mux2/1 -> Convert Attitude to UV coords./2
  Attitude Cmd./1 -> zoh/1
  v Control Law/1(Jet Command) -> Mux3/2  "v Jets"
  u Control Law/1(Jet Command) -> Mux3/1  "u Jets"
  Demux3/2 -> v Control Law/1(Position)  "v"
  Demux2/1 -> u Control Law/2(Rate)
  Demux1/1 -> [Yaw_error]  "Yaw error"
  Demux2/2 -> v Control Law/2(Rate)
  Mux3/1 -> Convert u,v to q,r coords./2
  u,v to q,r conversion matrix/1 -> Convert u,v to q,r coords./1
  Convert u,v to q,r coords./1 -> Pitch/Roll Jets/1  "Pitch and Roll Jets"
  Demux3/1 -> u Control Law/1(Position)  "u"

== system Final_Project_EEM_Particle_SIM/Reaction Jet Control/Reaction Jet Control_Accel ==
  Accel Cmd. : Inport  Unit=ft/sec^2
  Accel Meas. : Inport  Port=2  Unit=ft/sec^2
  Demux : Demux  Outputs=3
  Demux1 : Demux  Outputs=3
  Sum : Sum  Inputs=+-|  InputSameDT=on  SaturateOnIntegerOverflow=on  OutDataTypeStr=Inherit: Same as first input
  Sum1 : Sum  Inputs=+-|  InputSameDT=on  SaturateOnIntegerOverflow=on  OutDataTypeStr=Inherit: Same as first input
  Sum2 : Sum  Inputs=+-|  InputSameDT=on  SaturateOnIntegerOverflow=on  OutDataTypeStr=Inherit: Same as first input
  Zero-Order Hold at delt : ZeroOrderHold  SampleTime=delt
  Zero-Order Hold at delt1 : ZeroOrderHold  SampleTime=delt
  Zero-Order Hold at delt2 : ZeroOrderHold  SampleTime=delt
  zoh : ZeroOrderHold  SampleTime=delt
  zoh1 : ZeroOrderHold  SampleTime=delt
  zoh2 : ZeroOrderHold  SampleTime=delt
  Xaxis_accel : Outport  Unit=lbf  OutputWhenDisabled=reset  InitialOutput=0  VectorParamsAs1DForOutWhenUnconnected=off
  Yaxis_accel : Outport  Port=2  Unit=lbf  OutputWhenDisabled=reset  InitialOutput=0  VectorParamsAs1DForOutWhenUnconnected=off
  Zaxis_accel : Outport  Port=3  Unit=lbf  OutputWhenDisabled=reset  InitialOutput=0  VectorParamsAs1DForOutWhenUnconnected=off
  wires:
  zoh/1 -> Sum/2
  Accel Meas./1 -> Demux/1
  Sum2/1 -> Zaxis_accel/1  "Z accel Error"
  Accel Cmd./1 -> Demux1/1
  Sum/1 -> Xaxis_accel/1  "X accel error"
  Sum1/1 -> Yaxis_accel/1  "Y accel error"
  Demux/1 -> Zero-Order Hold at delt/1
  Demux/3 -> Zero-Order Hold at delt1/1
  Demux/2 -> Zero-Order Hold at delt2/1
  Zero-Order Hold at delt/1 -> Sum/1
  Demux1/1 -> zoh/1
  Demux1/2 -> zoh1/1
  Demux1/3 -> zoh2/1
  Zero-Order Hold at delt2/1 -> Sum1/1
  zoh1/1 -> Sum1/2
  zoh2/1 -> Sum2/2
  Zero-Order Hold at delt1/1 -> Sum2/1

== system Final_Project_EEM_Particle_SIM/Simulink 3D Animation/Convert to VR Units ==
  Att : Inport
  Pos : Inport  Port=2
  "LSAM Initial Offset " : Constant  Value=[-1.45132e+06 -1.13879e+06 -37269.6]
  Length Conversion : aerolibconvert2/Length Conversion  IU=ft  OU=m
  Rotation Matrix to VR Rotation : vrlib/Utilities/Rotation Matrix to VR Rotation  maxzero=1e-12
      settings: SourceProductBaseCode=SL
  Subtract : Sum  Inputs=+-
  attVR : Outport  VectorParamsAs1DForOutWhenUnconnected=off
  posVR : Outport  Port=2  VectorParamsAs1DForOutWhenUnconnected=off
  wires:
  Att/1 -> Rotation Matrix to VR Rotation/1
  Rotation Matrix to VR Rotation/1 -> attVR/1
  Pos/1 -> Length Conversion/1
  Length Conversion/1 -> Subtract/1
  Subtract/1 -> posVR/1
  "LSAM Initial Offset "/1 -> Subtract/2

== system Final_Project_EEM_Particle_SIM/Lunar Module Dynamics/6DOF ECEF (Quaternion)1/Angle Conversion ==
  in : Inport  Unit=deg
  Unit Conversion : UnitConversion
  out : Outport  Unit=rad  VectorParamsAs1DForOutWhenUnconnected=off
  wires:
  in/1 -> Unit Conversion/1
  Unit Conversion/1 -> out/1

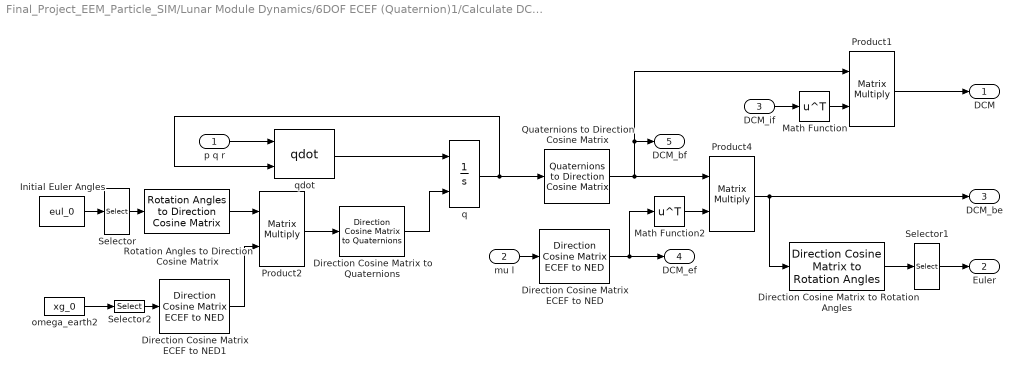
== system Final_Project_EEM_Particle_SIM/Lunar Module Dynamics/6DOF ECEF (Quaternion)1/Calculate DCM & Euler Angles ==
  p q r : Inport
  mu l : Inport  Port=2
  DCM_if : Inport  Port=3  PortDimensions=[3 3]
  Direction Cosine Matrix ECEF to NED : aerolibtransform2/Direction Cosine Matrix ECEF to NED
      settings: SourceProductBaseCode=AE
  Direction Cosine Matrix ECEF to NED1 : aerolibtransform2/Direction Cosine Matrix ECEF to NED
      settings: SourceProductBaseCode=AE
  Direction Cosine Matrix to Rotation Angles : sharedtransform/Direction Cosine Matrix to Rotation Angles  rotationOrder=ZYX  aMode=aMode  action=None  tolerance=eps(2)
      settings: SourceProductBaseCode=AE,PW,MT,VE,VP
  Direction Cosine Matrix to Quaternions : sharedtransform/Direction Cosine Matrix  to Quaternions  aMode=0  action=None  tolerance=eps(2)
      settings: SourceProductBaseCode=AE,PW,MT,VE,VP
  Initial Euler Angles : Constant  Value=eul_0
  Math Function : Math  Operator=transpose  SignedPower=on  SaturateOnIntegerOverflow=on
  Math Function2 : Math  Operator=transpose  SignedPower=on  SaturateOnIntegerOverflow=on
  Product1 : Product  Multiplication=Matrix(*)  RndMeth=Zero
  Product2 : Product  Multiplication=Matrix(*)  RndMeth=Zero
  Product4 : Product  Multiplication=Matrix(*)  RndMeth=Zero
  Quaternions to Direction Cosine Matrix : sharedtransform/Quaternions to  Direction Cosine Matrix  aMode=aMode
      settings: SourceProductBaseCode=AE,PW,MT,VE,VP
  Rotation Angles to Direction Cosine Matrix : sharedtransform/Rotation Angles to Direction Cosine Matrix  rotationOrder=ZYX  aMode=aMode
      settings: SourceProductBaseCode=AE,PW,MT,VE,VP
  Selector : Selector  InputPortWidth=3  IndexOptions=Index vector (dialog)  Indices=[3 2 1]  OutputSizes=1
  Selector1 : Selector  InputPortWidth=3  IndexOptions=Index vector (dialog)  Indices=[3 2 1]  OutputSizes=1
  Selector2 : Selector  InputPortWidth=3  IndexOptions=Index vector (dialog)  Indices=[1 2]  OutputSizes=1
  omega_earth2 : Constant  Value=xg_0
  q : Integrator  InitialConditionSource=external  InitialCondition=[e0_0 e1_0 e2_0 e3_0]  ContinuousStateAttributes=quat_statename
  qdot : shared6dofsys/qdot  aMode=aMode
      settings: SourceProductBaseCode=AE,PW,MT,VE,VP
  DCM : Outport  VectorParamsAs1DForOutWhenUnconnected=off
  Euler : Outport  Port=2  VectorParamsAs1DForOutWhenUnconnected=off
  DCM_be : Outport  Port=3  VectorParamsAs1DForOutWhenUnconnected=off
  DCM_ef : Outport  Port=4  VectorParamsAs1DForOutWhenUnconnected=off
  DCM_bf : Outport  Port=5  VectorParamsAs1DForOutWhenUnconnected=off
  wires:
  Selector1/1 -> Euler/1
  DCM_if/1 -> Math Function/1
  Direction Cosine Matrix ECEF to NED/1 -> DCM_ef/1, Math Function2/1
  Math Function/1 -> Product1/2
  p q r/1 -> qdot/1
  qdot/1 -> q/1
  Direction Cosine Matrix to Quaternions/1 -> q/2
  q/1 -> qdot/2, Quaternions to Direction Cosine Matrix/1
  Quaternions to Direction Cosine Matrix/1 -> Product1/1, DCM_bf/1, Product4/1
  Math Function2/1 -> Product4/2
  Product4/1 -> Direction Cosine Matrix to Rotation Angles/1, DCM_be/1
  Direction Cosine Matrix to Rotation Angles/1 -> Selector1/1
  Rotation Angles to Direction Cosine Matrix/1 -> Product2/1
  Product2/1 -> Direction Cosine Matrix to Quaternions/1
  Direction Cosine Matrix ECEF to NED1/1 -> Product2/2
  mu l/1 -> Direction Cosine Matrix ECEF to NED/1
  Product1/1 -> DCM/1
  Initial Euler Angles/1 -> Selector/1
  Selector/1 -> Rotation Angles to Direction Cosine Matrix/1
  omega_earth2/1 -> Selector2/1
  Selector2/1 -> Direction Cosine Matrix ECEF to NED1/1

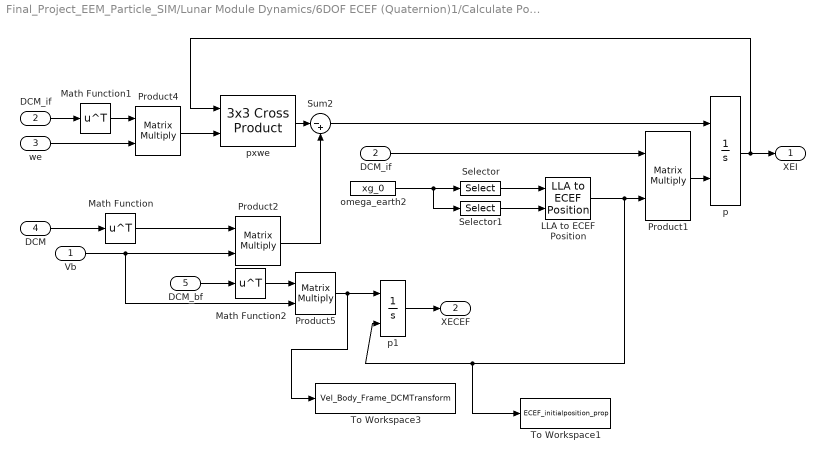
== system Final_Project_EEM_Particle_SIM/Lunar Module Dynamics/6DOF ECEF (Quaternion)1/Calculate Position in EI  ==
  Vb : Inport
  DCM_if : Inport  Port=2
  we : Inport  Port=3
  DCM : Inport  Port=4
  DCM_bf : Inport  Port=5
  "DCM_if " : InportShadow  Port=2
  LLA to ECEF Position : aerolibtransform2/LLA to ECEF Position  units=Metric (MKS)  ptype=Custom  F=F  R=R
      settings: SourceProductBaseCode=AE
  Math Function : Math  Operator=transpose  SignedPower=on  SaturateOnIntegerOverflow=on
  Math Function1 : Math  Operator=transpose  SignedPower=on  SaturateOnIntegerOverflow=on
  Math Function2 : Math  Operator=transpose  SignedPower=on  SaturateOnIntegerOverflow=on
  Product{1..2,4..5} (4 alike) : Product  Multiplication=Matrix(*)  RndMeth=Zero
  Selector : Selector  InputPortWidth=3  IndexOptions=Index vector (dialog)  Indices=[1 2]  OutputSizes=1
  Selector1 : Selector  InputPortWidth=3  IndexOptions=Index vector (dialog)  Indices=[3]  OutputSizes=1
  Sum2 : Sum  Inputs=|-+  SaturateOnIntegerOverflow=on
  To Workspace1 : ToWorkspace  VariableName=ECEF_initialposition_prop  SampleTime=0.1
      settings: Save2DSignal=2-D array (concatenate along first dimension)
  To Workspace3 : ToWorkspace  VariableName=Vel_Body_Frame_DCMTransform  SampleTime=0.1
      settings: Save2DSignal=2-D array (concatenate along first dimension)
  omega_earth2 : Constant  Value=xg_0
  p : Integrator  InitialConditionSource=external  ContinuousStateAttributes=posECI_statename
  p1 : Integrator  InitialConditionSource=external  ContinuousStateAttributes=posECEF_statename
  pxwe : sharedutil/3x3 Cross Product  aMode=aMode
      settings: SourceProductBaseCode=AE,PW,MT,VE,VP
  XEI : Outport  VectorParamsAs1DForOutWhenUnconnected=off
  XECEF : Outport  Port=2  VectorParamsAs1DForOutWhenUnconnected=off
  wires:
  Math Function2/1 -> Product5/1
  DCM_bf/1 -> Math Function2/1
  Math Function1/1 -> Product4/1
  "DCM_if "/1 -> Math Function1/1
  Product4/1 -> pxwe/2
  p/1 -> XEI/1, pxwe/1
  we/1 -> Product4/2
  Product2/1 -> Sum2/2
  DCM/1 -> Math Function/1
  DCM_if/1 -> Product1/1
  p1/1 -> XECEF/1
  Math Function/1 -> Product2/1
  Vb/1 -> Product2/2, Product5/2
  Product5/1 -> To Workspace3/1, p1/1
  Sum2/1 -> p/1
  LLA to ECEF Position/1 -> Product1/2, To Workspace1/1, p1/2
  Product1/1 -> p/2
  pxwe/1 -> Sum2/1
  Selector/1 -> LLA to ECEF Position/1
  Selector1/1 -> LLA to ECEF Position/2
  omega_earth2/1 -> Selector1/1, Selector/1

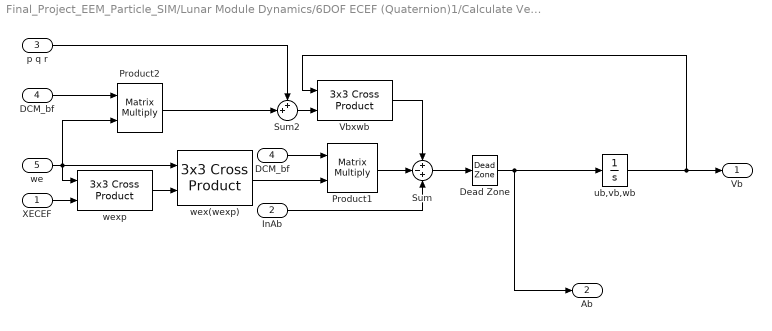
== system Final_Project_EEM_Particle_SIM/Lunar Module Dynamics/6DOF ECEF (Quaternion)1/Calculate Velocity in Body Axes ==
  XECEF : Inport
  InAb : Inport  Port=2
  p q r : Inport  Port=3
  DCM_bf : Inport  Port=4
  we : Inport  Port=5
  "DCM_bf " : InportShadow  Port=4
  Dead Zone : DeadZone  LowerValue=-eps  UpperValue=eps  SaturateOnIntegerOverflow=on
  Product1 : Product  Multiplication=Matrix(*)  RndMeth=Zero
  Product2 : Product  Multiplication=Matrix(*)  RndMeth=Zero
  Sum : Sum  Inputs=+-+  SaturateOnIntegerOverflow=on
  Sum2 : Sum  Inputs=++|  SaturateOnIntegerOverflow=on
  Vbxwb : sharedutil/3x3 Cross Product  aMode=aMode
      settings: SourceProductBaseCode=AE,PW,MT,VE,VP
  ub,vb,wb : Integrator  InitialCondition=Vm_0  ContinuousStateAttributes=Vm_statename
  wex(wexp) : sharedutil/3x3 Cross Product  aMode=aMode
      settings: SourceProductBaseCode=AE,PW,MT,VE,VP
  wexp : sharedutil/3x3 Cross Product  aMode=aMode
      settings: SourceProductBaseCode=AE,PW,MT,VE,VP
  Vb : Outport  VectorParamsAs1DForOutWhenUnconnected=off
  Ab : Outport  Port=2  PortDimensions=3  VectorParamsAs1DForOutWhenUnconnected=off
  wires:
  DCM_bf/1 -> Product1/1
  we/1 -> wex(wexp)/1, wexp/1, Product2/2
  InAb/1 -> Sum/3
  Vbxwb/1 -> Sum/1
  XECEF/1 -> wexp/2
  wex(wexp)/1 -> Product1/2
  wexp/1 -> wex(wexp)/2
  Product2/1 -> Sum2/2
  Sum2/1 -> Vbxwb/2
  Product1/1 -> Sum/2
  Sum/1 -> Dead Zone/1
  ub,vb,wb/1 -> Vbxwb/1, Vb/1
  "DCM_bf "/1 -> Product2/1
  p q r/1 -> Sum2/1
  Dead Zone/1 -> ub,vb,wb/1, Ab/1

== system Final_Project_EEM_Particle_SIM/Lunar Module Dynamics/6DOF ECEF (Quaternion)1/Celestial Longitude of Greenwich ==
  Initial Angle : Inport  Unit=rad
  Constant1 : Constant  Value=w_E
  Integrator : Integrator  ContinuousStateAttributes=LG_statename
  Sum : Sum  Inputs=|++
  Lambda : Outport  VectorParamsAs1DForOutWhenUnconnected=off
  wires:
  Initial Angle/1 -> Sum/1
  Integrator/1 -> Sum/2
  Constant1/1 -> Integrator/1  "we"
  Sum/1 -> Lambda/1

== system Final_Project_EEM_Particle_SIM/Lunar Module Dynamics/6DOF ECEF (Quaternion)1/ECEF to Inertial ==
  LG : Inport
  Create 3x3 Matrix : sharedutil/Create 3x3 Matrix  aMode=aMode
      settings: SourceProductBaseCode=AE,PW,MT,VE,VP
  Unary Minus : UnaryMinus
  Zero : Constant  Value=0
  Zero1 : Constant
  sincos : Trigonometry  Operator=sincos
  DCM_IF : Outport  VectorParamsAs1DForOutWhenUnconnected=off
  wires:
  LG/1 -> sincos/1
  Create 3x3 Matrix/1 -> DCM_IF/1
  Zero1/1 -> Create 3x3 Matrix/9
  Zero/1 -> Create 3x3 Matrix/8, Create 3x3 Matrix/7, Create 3x3 Matrix/6, Create 3x3 Matrix/3
  sincos/2 -> Create 3x3 Matrix/1, Create 3x3 Matrix/5
  sincos/1 -> Create 3x3 Matrix/4, Unary Minus/1
  Unary Minus/1 -> Create 3x3 Matrix/2

== system Final_Project_EEM_Particle_SIM/Lunar Module Dynamics/6DOF ECEF (Quaternion)1/Velocity Conversion ==
  in : Inport  Unit=ft/s
  Unit Conversion : UnitConversion
  out : Outport  VectorParamsAs1DForOutWhenUnconnected=off
  wires:
  in/1 -> Unit Conversion/1
  Unit Conversion/1 -> out/1

== system Final_Project_EEM_Particle_SIM/Lunar Module Dynamics/6DOF ECEF (Quaternion)1/Velocity Conversion1 ==
  in : Inport  Unit=ft/sec^2
  Unit Conversion : UnitConversion
  out : Outport  VectorParamsAs1DForOutWhenUnconnected=off
  wires:
  in/1 -> Unit Conversion/1
  Unit Conversion/1 -> out/1
